simulink model "fullsteeringmodel"  (R2024b)
settings: Solver=VariableStepAuto  StartTime=0.0  StopTime=10.0  RelTol=1e-3
settings Model: Creator=rober  LastModifiedBy=rober

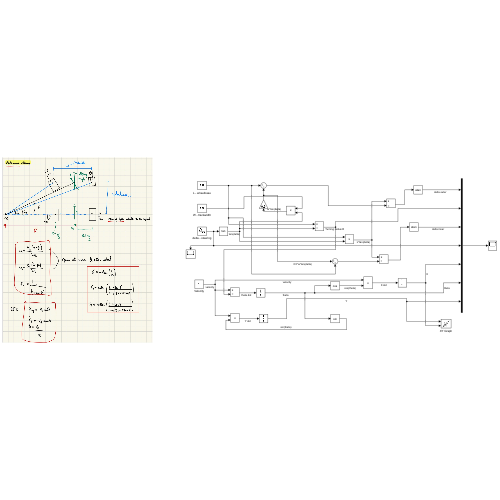
[thumbnail: Simulink's stored preview of the top-level diagram]
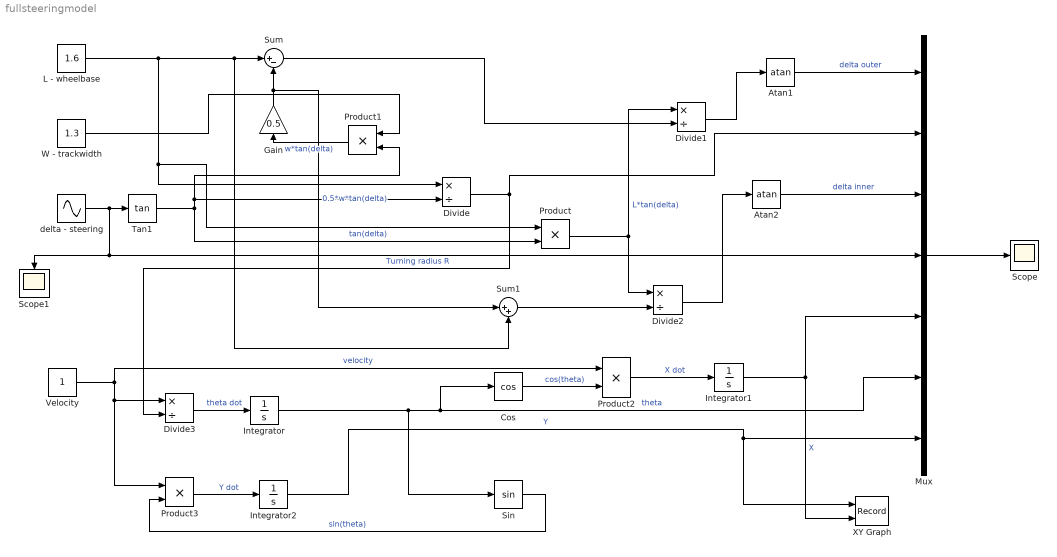
== system fullsteeringmodel ==
  Atan1 : Trigonometry  Operator=atan
  Atan2 : Trigonometry  Operator=atan
  Cos : Trigonometry  Operator=cos
  Divide{,1..3} (4 alike) : Product  Inputs=*/
  Gain : Gain  Gain=0.5
  Integrator : Integrator
  Integrator1 : Integrator
  Integrator2 : Integrator
  L - wheelbase : Constant  Value=1.6
  Mux : Mux  Inputs=7
  Product{,1..3} (4 alike) : Product
  Scope : Scope
  Scope1 : Scope
  Sin : Trigonometry
  Sum : Sum  Inputs=|+-
  Sum1 : Sum  Inputs=|++
  Tan1 : Trigonometry  Operator=tan
  Velocity : Constant
  W - trackwidth : Constant  Value=1.3
  XY Graph : Record  FileSettingsInternal="{\"entries\":[{\"content\":{\"excelSettings\":{\"content\":{},\"type\":\"Streamout.ExcelSettings\"}},\"type\":\"Streamout.FileSettingStorage\",\"uuid\":\"\"}],\"packageUris\":[\"http:\\/\\/schema.mathworks.com\\/mf0\\/streamout_blocks\\/R2020a\"],\"version\":\"1.0\"}"  Layout=[1 1]  SignalsInternal="{\"entries\":[{\"content\":{\"signals\":[{\"content\":{\"blockPath\":[],\"dimensions\":[1],\"domain\":\"\",\"lineColor\":\"#a2142f\",\"plots\":[ 1 ],\"port\":1,\"signalID\":1,\"signalName\":\"Y\"},\"type\":\"RecordBlkView.Signal\",\"uuid\":\"\"},{\"content\":{\"blockPath\":[],\"dimensions\":[1],\"domain\":\"\",\"lineColor\":\"#139fff\",\"plots\":[ 1 ],\"port\":2,\"signalID\":2,\"signalName\":\"X\"},\"type\":\"RecordBlkView.Signal\",\"uuid\":\"\"}]},\"type\":\"RecordBlkView.InputSignals\",\"uuid\":\"\"}],\"packageUris\":[\"http:\\/\\/schema.mathworks.com\\/mf0\\/streamout_blocks\\/R2020a\"],\"version\":\"1.0\"}"  VisualizationBindings="{\"xyplotplugin\":{\"info\":[{\"series\":[{\"bindingParametersList\":[{\"parameter\":\"X-Axis\",\"signalID\":1,\"signalName\":\"Y\"},{\"parameter\":\"Y-Axis\",\"signalID\":2,\"signalName\":\"X\"}],\"seriesID\":0}],\"subplotID\":1}]}}"  CompatibilityTag=XY
  delta - steering : Sin  Phase=0.1  SampleTime=0
  wires:
  delta - steering/1 -> Scope1/1, Mux/4, Tan1/1
  L - wheelbase/1 -> Sum1/2, Sum/1, Product/1, Divide/1
  Divide/1 -> Divide3/2, Mux/2  "Turning radius R"
  Gain/1 -> Sum1/1, Sum/2  "0.5*w*tan(delta)"
  W - trackwidth/1 -> Product1/1
  Product1/1 -> Gain/1  "w*tan(delta)"
  Sum/1 -> Divide1/2
  Product/1 -> Divide1/1, Divide2/1  "L*tan(delta)"
  Divide1/1 -> Atan1/1
  Atan1/1 -> Mux/1  "delta outer"
  Mux/1 -> Scope/1
  Sum1/1 -> Divide2/2
  Divide2/1 -> Atan2/1
  Atan2/1 -> Mux/3  "delta inner"
  Velocity/1 -> Product3/1, Divide3/1, Product2/1  "velocity"
  Divide3/1 -> Integrator/1  "theta dot"
  Integrator/1 -> Sin/1, Mux/6, Cos/1  "theta"
  Tan1/1 -> Product1/2, Divide/2, Product/2  "tan(delta)"
  Cos/1 -> Product2/2  "cos(theta)"
  Product2/1 -> Integrator1/1  "X dot"
  Integrator1/1 -> XY Graph/2, Mux/5  "X"
  Sin/1 -> Product3/2  "sin(theta)"
  Product3/1 -> Integrator2/1  "Y dot"
  Integrator2/1 -> XY Graph/1, Mux/7  "Y"
